simulink model "simulare"  (R2025b)
settings: Solver=VariableStepAuto  StartTime=0.0  StopTime=5  MaxStep=0.01  RelTol=1e-3
libraries: simulink x9
settings Model: Creator=alexolaru131  LastModifiedBy=alexolaru131

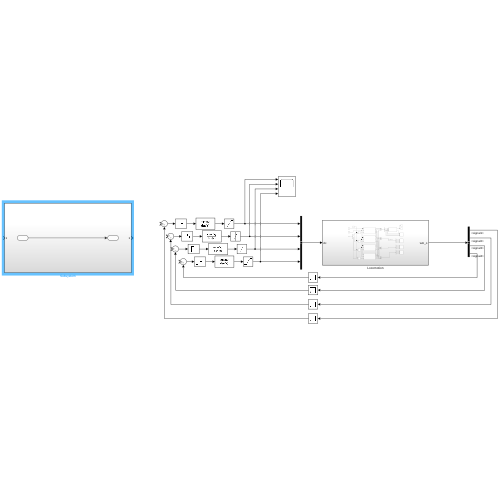
[thumbnail: Simulink's stored preview of the top-level diagram]
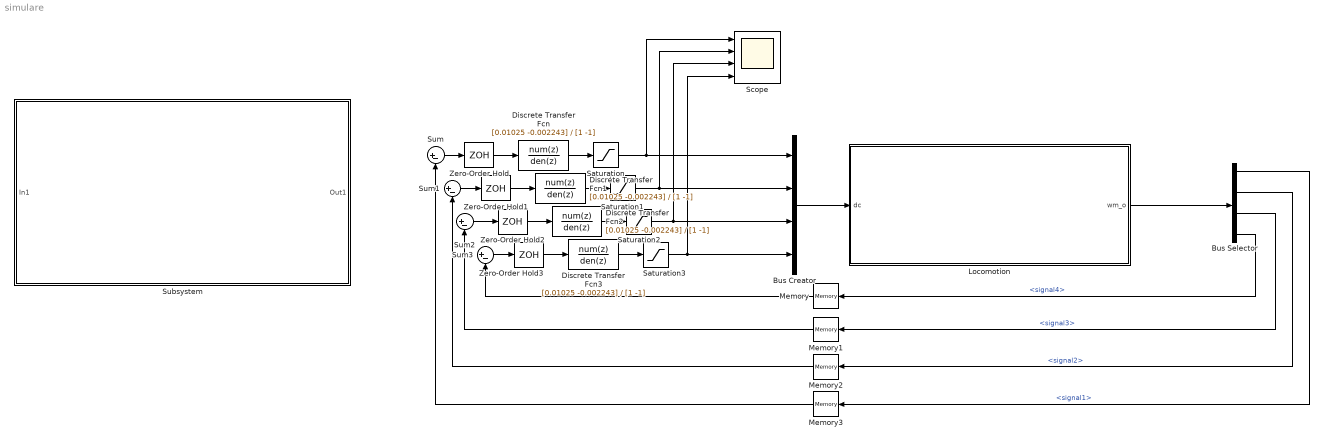
== system simulare ==
  Bus Creator : BusCreator  Inputs=4
  Bus Selector : BusSelector  OutputSignals=signal1,signal2,signal3,signal4
  Discrete Transfer Fcn{,1..3} (4 alike) : DiscreteTransferFcn  Numerator=[0.01025 -0.002243]  Denominator=[1 -1]
  Locomotion : Subsystem
  Memory{,1..3} (4 alike) : Memory
  Saturation{,1..3} (4 alike) : Saturate  UpperLimit=1  LowerLimit=0
  Scope : Scope  NumInputPorts=4
      settings: ActiveDisplayYMinimum=-1  ActiveDisplayYMaximum=1  DataLoggingVariableName=ScopeData4
  Subsystem : Subsystem
  Sum{,1..3} (4 alike) : Sum  Inputs=|+-
  Zero-Order Hold{,1..3} (4 alike) : ZeroOrderHold  SampleTime=0.1
  wires:
  Zero-Order Hold/1 -> Discrete Transfer Fcn/1
  Discrete Transfer Fcn/1 -> Saturation/1
  Sum/1 -> Zero-Order Hold/1
  Locomotion/1(wm_o) -> Bus Selector/1
  Bus Selector/1 -> Memory3/1  "<signal1>"
  Saturation/1 -> Scope/1, Bus Creator/1
  Saturation1/1 -> Bus Creator/2, Scope/2
  Discrete Transfer Fcn1/1 -> Saturation1/1
  Sum1/1 -> Zero-Order Hold1/1
  Zero-Order Hold1/1 -> Discrete Transfer Fcn1/1
  Bus Selector/2 -> Memory2/1  "<signal2>"
  Discrete Transfer Fcn2/1 -> Saturation2/1
  Zero-Order Hold2/1 -> Discrete Transfer Fcn2/1
  Saturation2/1 -> Bus Creator/3, Scope/3
  Sum2/1 -> Zero-Order Hold2/1
  Bus Selector/3 -> Memory1/1  "<signal3>"
  Discrete Transfer Fcn3/1 -> Saturation3/1
  Zero-Order Hold3/1 -> Discrete Transfer Fcn3/1
  Sum3/1 -> Zero-Order Hold3/1
  Saturation3/1 -> Bus Creator/4, Scope/4
  Bus Selector/4 -> Memory/1  "<signal4>"
  Memory/1 -> Sum3/2
  Memory1/1 -> Sum2/2
  Memory2/1 -> Sum1/2
  Memory3/1 -> Sum/2
  Bus Creator/1 -> Locomotion/1(dc)

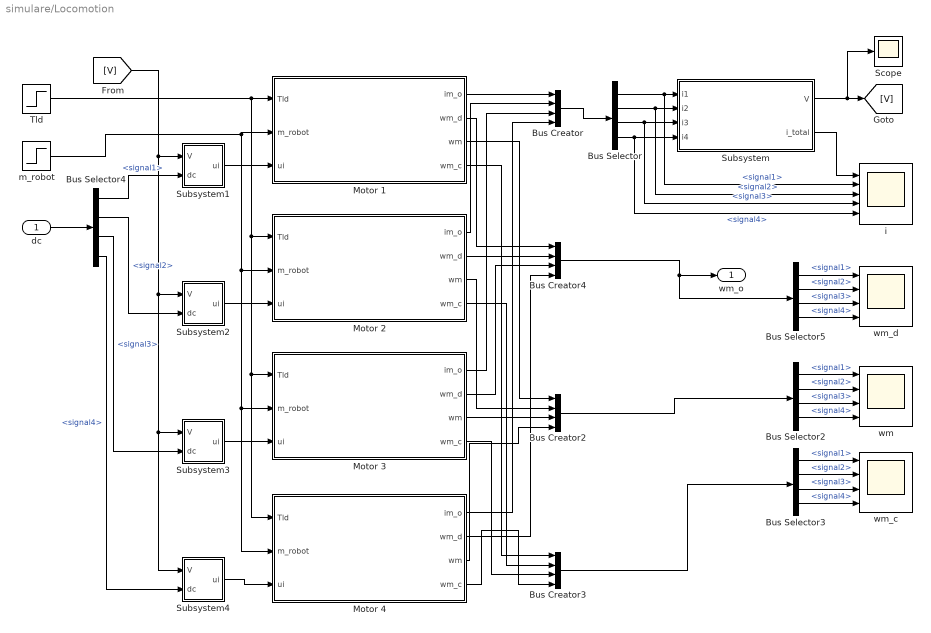
== system simulare/Locomotion ==
  dc : Inport
  Bus Creator{,2..4} (4 alike) : BusCreator  Inputs=4
  Bus Selector{,2..5} (5 alike) : BusSelector  OutputSignals=signal1,signal2,signal3,signal4
  Motor 1 : Subsystem
  Motor 2 : Subsystem
  Motor 3 : Subsystem
  Motor 4 : Subsystem
  Scope : Scope
      settings: ActiveDisplayYMinimum=-1  ActiveDisplayYMaximum=1
  Subsystem : Subsystem
  Subsystem1 : Subsystem
  Subsystem2 : Subsystem
  Subsystem3 : Subsystem
  Subsystem4 : Subsystem
  Tld : Step  Time=0  After=0.5  SampleTime=0
  i : Scope  NumInputPorts=5
      settings: ActiveDisplayYMinimum=-0.41798303299260658  ActiveDisplayYMaximum=3.1723127947753986
  m_robot : Step  Time=0  After=2000  SampleTime=0
  wm : Scope  NumInputPorts=4
      settings: ActiveDisplayYMinimum=-2.7499999999999996  ActiveDisplayYMaximum=24.75
  wm_c : Scope  NumInputPorts=4
      settings: ActiveDisplayYMinimum=-3.6972275501307741  ActiveDisplayYMaximum=33.275047951176973  DataLoggingVariableName=ScopeData3
  wm_d : Scope  NumInputPorts=4
      settings: ActiveDisplayYMinimum=-3.9543093339999862  ActiveDisplayYMaximum=35.588776352959464  DataLoggingVariableName=ScopeData2
  wm_o : Outport
  wires:
  Subsystem2/1(ui) -> Motor 2/3(ui)
  Subsystem1/1(ui) -> Motor 1/3(ui)
  Subsystem/2(i_total) -> i/1
  m_robot/1 -> Motor 1/2(m_robot), Motor 2/2(m_robot), Motor 3/2(m_robot), Motor 4/2(m_robot)
  Subsystem4/1(ui) -> Motor 4/3(ui)
  Tld/1 -> Motor 1/1(Tld), Motor 2/1(Tld), Motor 3/1(Tld), Motor 4/1(Tld)
  Subsystem3/1(ui) -> Motor 3/3(ui)
  Bus Creator/1 -> Bus Selector/1
  Bus Selector/1 -> i/2, Subsystem/1(i1)  "<signal1>"
  Bus Selector/2 -> Subsystem/2(i2), i/3  "<signal2>"
  Bus Selector/3 -> Subsystem/3(i3), i/4  "<signal3>"
  Bus Selector/4 -> Subsystem/4(i4), i/5  "<signal4>"
  Subsystem/1(V) -> Scope/1, [V]
  [V] -> Subsystem1/1(V), Subsystem2/1(V), Subsystem3/1(V), Subsystem4/1(V)
  Bus Selector2/2 -> wm/2  "<signal2>"
  Bus Selector2/1 -> wm/1  "<signal1>"
  Bus Selector2/3 -> wm/3  "<signal3>"
  Bus Selector2/4 -> wm/4  "<signal4>"
  Bus Creator2/1 -> Bus Selector2/1
  Bus Selector3/1 -> wm_c/1  "<signal1>"
  Bus Selector3/2 -> wm_c/2  "<signal2>"
  Bus Selector3/3 -> wm_c/3  "<signal3>"
  Bus Selector3/4 -> wm_c/4  "<signal4>"
  Bus Creator3/1 -> Bus Selector3/1
  Bus Selector5/4 -> wm_d/4  "<signal4>"
  Bus Creator4/1 -> Bus Selector5/1, wm_o/1
  Bus Selector5/2 -> wm_d/2  "<signal2>"
  Bus Selector5/3 -> wm_d/3  "<signal3>"
  Bus Selector5/1 -> wm_d/1  "<signal1>"
  Bus Selector4/1 -> Subsystem1/2(dc)  "<signal1>"
  Bus Selector4/2 -> Subsystem2/2(dc)  "<signal2>"
  Bus Selector4/3 -> Subsystem3/2(dc)  "<signal3>"
  Bus Selector4/4 -> Subsystem4/2(dc)  "<signal4>"
  dc/1 -> Bus Selector4/1
  Motor 1/1(im_o) -> Bus Creator/1
  Motor 2/1(im_o) -> Bus Creator/2
  Motor 3/1(im_o) -> Bus Creator/3
  Motor 4/1(im_o) -> Bus Creator/4
  Motor 1/2(wm_d) -> Bus Creator4/1
  Motor 2/2(wm_d) -> Bus Creator4/2
  Motor 3/2(wm_d) -> Bus Creator4/3
  Motor 4/2(wm_d) -> Bus Creator4/4
  Motor 1/3(wm) -> Bus Creator2/1
  Motor 2/3(wm) -> Bus Creator2/2
  Motor 3/3(wm) -> Bus Creator2/3
  Motor 4/3(wm) -> Bus Creator2/4
  Motor 1/4(wm_c) -> Bus Creator3/1
  Motor 2/4(wm_c) -> Bus Creator3/2
  Motor 3/4(wm_c) -> Bus Creator3/3
  Motor 4/4(wm_c) -> Bus Creator3/4

== system simulare/Subsystem ==
  In1 : Inport
  Out1 : Outport
  wires:
  In1/1 -> Out1/1

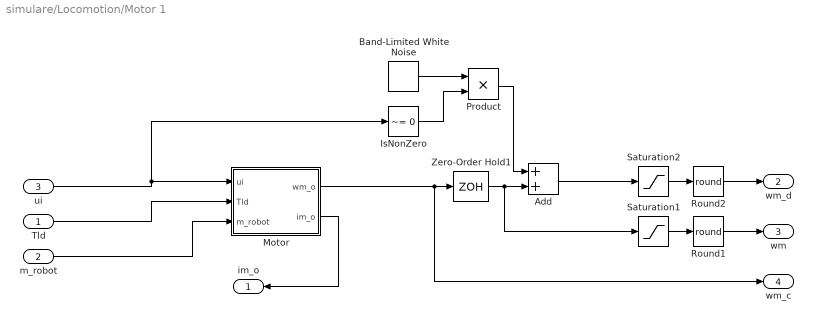
== system simulare/Locomotion/Motor 1 ==
  Tld : Inport
  m_robot : Inport  Port=2
  ui : Inport  Port=3
  Add : Sum
  Band-Limited White Noise : simulink/Sources/Band-Limited White Noise  Cov=[0.2]  Ts=0.1  seed=[1]
  IsNonZero : simulink/Logic and Bit Operations/Compare To Zero  relop=~=  OutDataTypeStr=boolean
      settings: LibrarySourceBlock=|
      | simulink/Quick Insert/Logic and Bit
      | Operations/IsNonZero
  Motor : Subsystem
  Product : Product
  Round1 : Rounding  Operator=round
  Round2 : Rounding  Operator=round
  Saturation1 : Saturate  UpperLimit=inf  LowerLimit=0
  Saturation2 : Saturate  UpperLimit=inf  LowerLimit=0
  Zero-Order Hold1 : ZeroOrderHold  SampleTime=0.1
  im_o : Outport
  wm_d : Outport  Port=2
  wm : Outport  Port=3
  wm_c : Outport  Port=4
  wires:
  Motor/2(im_o) -> im_o/1
  Tld/1 -> Motor/2(Tld)
  m_robot/1 -> Motor/3(m_robot)
  ui/1 -> IsNonZero/1, Motor/1(ui)
  Motor/1(wm_o) -> wm_c/1, Zero-Order Hold1/1
  IsNonZero/1 -> Product/2
  Product/1 -> Add/1
  Add/1 -> Saturation2/1
  Zero-Order Hold1/1 -> Saturation1/1, Add/2
  Saturation1/1 -> Round1/1
  Round1/1 -> wm/1
  Band-Limited White Noise/1 -> Product/1
  Round2/1 -> wm_d/1
  Saturation2/1 -> Round2/1

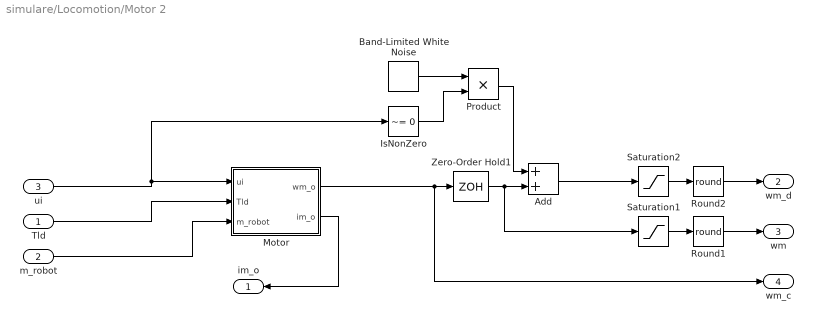
== system simulare/Locomotion/Motor 2 ==
  Tld : Inport
  m_robot : Inport  Port=2
  ui : Inport  Port=3
  Add : Sum
  Band-Limited White Noise : simulink/Sources/Band-Limited White Noise  Cov=[0.2]  Ts=0.1  seed=[2]
  IsNonZero : simulink/Logic and Bit Operations/Compare To Zero  relop=~=  OutDataTypeStr=boolean
      settings: LibrarySourceBlock=|
      | simulink/Quick Insert/Logic and Bit
      | Operations/IsNonZero
  Motor : Subsystem
  Product : Product
  Round1 : Rounding  Operator=round
  Round2 : Rounding  Operator=round
  Saturation1 : Saturate  UpperLimit=inf  LowerLimit=0
  Saturation2 : Saturate  UpperLimit=inf  LowerLimit=0
  Zero-Order Hold1 : ZeroOrderHold  SampleTime=0.1
  im_o : Outport
  wm_d : Outport  Port=2
  wm : Outport  Port=3
  wm_c : Outport  Port=4
  wires:
  Motor/2(im_o) -> im_o/1
  Tld/1 -> Motor/2(Tld)
  m_robot/1 -> Motor/3(m_robot)
  ui/1 -> IsNonZero/1, Motor/1(ui)
  Motor/1(wm_o) -> wm_c/1, Zero-Order Hold1/1
  IsNonZero/1 -> Product/2
  Product/1 -> Add/1
  Add/1 -> Saturation2/1
  Zero-Order Hold1/1 -> Saturation1/1, Add/2
  Saturation1/1 -> Round1/1
  Round1/1 -> wm/1
  Band-Limited White Noise/1 -> Product/1
  Round2/1 -> wm_d/1
  Saturation2/1 -> Round2/1

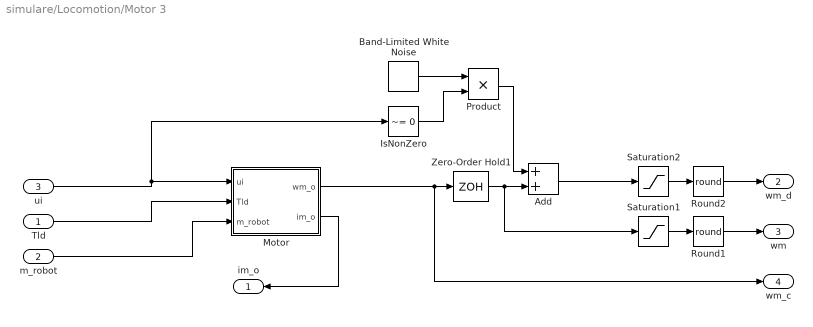
== system simulare/Locomotion/Motor 3 ==
  Tld : Inport
  m_robot : Inport  Port=2
  ui : Inport  Port=3
  Add : Sum
  Band-Limited White Noise : simulink/Sources/Band-Limited White Noise  Cov=[0.2]  Ts=0.1  seed=[3]
  IsNonZero : simulink/Logic and Bit Operations/Compare To Zero  relop=~=  OutDataTypeStr=boolean
      settings: LibrarySourceBlock=|
      | simulink/Quick Insert/Logic and Bit
      | Operations/IsNonZero
  Motor : Subsystem
  Product : Product
  Round1 : Rounding  Operator=round
  Round2 : Rounding  Operator=round
  Saturation1 : Saturate  UpperLimit=inf  LowerLimit=0
  Saturation2 : Saturate  UpperLimit=inf  LowerLimit=0
  Zero-Order Hold1 : ZeroOrderHold  SampleTime=0.1
  im_o : Outport
  wm_d : Outport  Port=2
  wm : Outport  Port=3
  wm_c : Outport  Port=4
  wires:
  Motor/2(im_o) -> im_o/1
  Tld/1 -> Motor/2(Tld)
  m_robot/1 -> Motor/3(m_robot)
  ui/1 -> IsNonZero/1, Motor/1(ui)
  Motor/1(wm_o) -> wm_c/1, Zero-Order Hold1/1
  IsNonZero/1 -> Product/2
  Product/1 -> Add/1
  Add/1 -> Saturation2/1
  Zero-Order Hold1/1 -> Saturation1/1, Add/2
  Saturation1/1 -> Round1/1
  Round1/1 -> wm/1
  Band-Limited White Noise/1 -> Product/1
  Round2/1 -> wm_d/1
  Saturation2/1 -> Round2/1

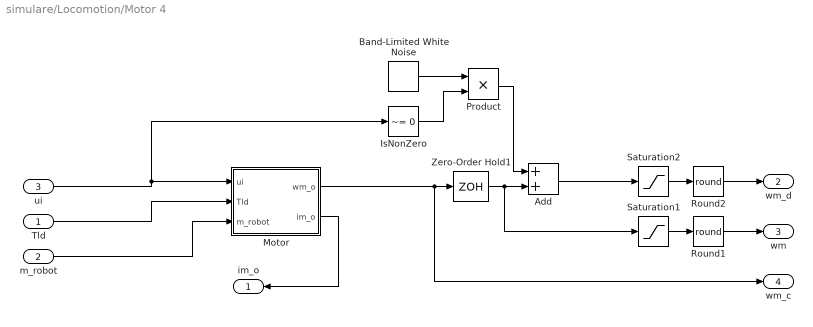
== system simulare/Locomotion/Motor 4 ==
  Tld : Inport
  m_robot : Inport  Port=2
  ui : Inport  Port=3
  Add : Sum
  Band-Limited White Noise : simulink/Sources/Band-Limited White Noise  Cov=[0.2]  Ts=0.1  seed=[4]
  IsNonZero : simulink/Logic and Bit Operations/Compare To Zero  relop=~=  OutDataTypeStr=boolean
      settings: LibrarySourceBlock=|
      | simulink/Quick Insert/Logic and Bit
      | Operations/IsNonZero
  Motor : Subsystem
  Product : Product
  Round1 : Rounding  Operator=round
  Round2 : Rounding  Operator=round
  Saturation1 : Saturate  UpperLimit=inf  LowerLimit=0
  Saturation2 : Saturate  UpperLimit=inf  LowerLimit=0
  Zero-Order Hold1 : ZeroOrderHold  SampleTime=0.1
  im_o : Outport
  wm_d : Outport  Port=2
  wm : Outport  Port=3
  wm_c : Outport  Port=4
  wires:
  Motor/2(im_o) -> im_o/1
  Tld/1 -> Motor/2(Tld)
  m_robot/1 -> Motor/3(m_robot)
  ui/1 -> IsNonZero/1, Motor/1(ui)
  Motor/1(wm_o) -> wm_c/1, Zero-Order Hold1/1
  IsNonZero/1 -> Product/2
  Product/1 -> Add/1
  Add/1 -> Saturation2/1
  Zero-Order Hold1/1 -> Saturation1/1, Add/2
  Saturation1/1 -> Round1/1
  Round1/1 -> wm/1
  Band-Limited White Noise/1 -> Product/1
  Round2/1 -> wm_d/1
  Saturation2/1 -> Round2/1

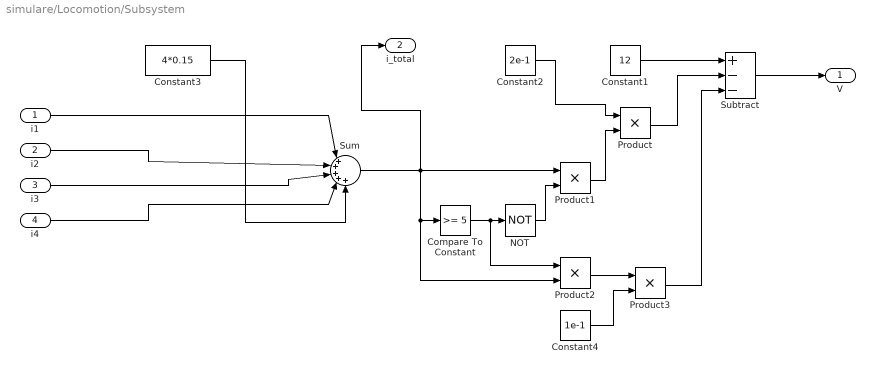
== system simulare/Locomotion/Subsystem ==
  i1 : Inport
  i2 : Inport  Port=2
  i3 : Inport  Port=3
  i4 : Inport  Port=4
  Compare To Constant : simulink/Logic and Bit Operations/Compare To Constant  relop=>=  const=5  OutDataTypeStr=boolean  ZeroCross=off
  Constant1 : Constant  Value=12
  Constant2 : Constant  Value=2e-1
  Constant3 : Constant  Value=4*0.15
  Constant4 : Constant  Value=1e-1
  NOT : Logic  Operator=NOT  IconShape=distinctive  AllPortsSameDT=off  OutDataTypeStr=boolean
  Product{,1..3} (4 alike) : Product
  Subtract : Sum  Inputs=+--
  Sum : Sum  Inputs=|+++++
  V : Outport
  i_total : Outport  Port=2
  wires:
  Constant2/1 -> Product/1
  Product/1 -> Subtract/2
  Sum/1 -> Product2/2, Compare To Constant/1, Product1/1, i_total/1
  Constant3/1 -> Sum/5
  Constant1/1 -> Subtract/1
  i1/1 -> Sum/1
  i2/1 -> Sum/2
  i3/1 -> Sum/3
  i4/1 -> Sum/4
  Subtract/1 -> V/1
  Compare To Constant/1 -> Product2/1, NOT/1
  NOT/1 -> Product1/2
  Product1/1 -> Product/2
  Product2/1 -> Product3/1
  Product3/1 -> Subtract/3
  Constant4/1 -> Product3/2

== system simulare/Locomotion/Subsystem1 ==
  V : Inport
  dc : Inport  Port=2
  Add : Sum  Inputs=+-
  Constant : Constant  Value=1.2782
  Product : Product
  ui : Outport
  wires:
  Add/1 -> Product/1
  V/1 -> Add/1
  dc/1 -> Product/2
  Constant/1 -> Add/2
  Product/1 -> ui/1

== system simulare/Locomotion/Subsystem2 ==
  V : Inport
  dc : Inport  Port=2
  Add : Sum  Inputs=+-
  Constant : Constant  Value=1.2782
  Product : Product
  ui : Outport
  wires:
  Add/1 -> Product/1
  V/1 -> Add/1
  dc/1 -> Product/2
  Constant/1 -> Add/2
  Product/1 -> ui/1

== system simulare/Locomotion/Subsystem3 ==
  V : Inport
  dc : Inport  Port=2
  Add : Sum  Inputs=+-
  Constant : Constant  Value=1.2782
  Product : Product
  ui : Outport
  wires:
  Add/1 -> Product/1
  V/1 -> Add/1
  dc/1 -> Product/2
  Constant/1 -> Add/2
  Product/1 -> ui/1

== system simulare/Locomotion/Subsystem4 ==
  V : Inport
  dc : Inport  Port=2
  Add : Sum  Inputs=+-
  Constant : Constant  Value=1.2782
  Product : Product
  ui : Outport
  wires:
  Add/1 -> Product/1
  V/1 -> Add/1
  dc/1 -> Product/2
  Constant/1 -> Add/2
  Product/1 -> ui/1

== system simulare/Locomotion/Motor 1/Motor ==
  ui : Inport
  Tld : Inport  Port=2
  m_robot : Inport  Port=3
  Electric : Subsystem
  Mecanic : Subsystem
  wm_o : Outport
  im_o : Outport  Port=2
  wires:
  Tld/1 -> Mecanic/2(Tld)
  Mecanic/1(wm_o) -> wm_o/1, Electric/3(wm), Mecanic/3(wm_i)
  Electric/1(im_o) -> im_o/1, Mecanic/1(im_i), Electric/2(im_i)
  m_robot/1 -> Mecanic/4(m_robot)
  ui/1 -> Electric/1(ui)

== system simulare/Locomotion/Motor 2/Motor ==
  ui : Inport
  Tld : Inport  Port=2
  m_robot : Inport  Port=3
  Electric : Subsystem
  Mecanic : Subsystem
  wm_o : Outport
  im_o : Outport  Port=2
  wires:
  Tld/1 -> Mecanic/2(Tld)
  Mecanic/1(wm_o) -> wm_o/1, Electric/3(wm), Mecanic/3(wm_i)
  Electric/1(im_o) -> im_o/1, Mecanic/1(im_i), Electric/2(im_i)
  m_robot/1 -> Mecanic/4(m_robot)
  ui/1 -> Electric/1(ui)

== system simulare/Locomotion/Motor 3/Motor ==
  ui : Inport
  Tld : Inport  Port=2
  m_robot : Inport  Port=3
  Electric : Subsystem
  Mecanic : Subsystem
  wm_o : Outport
  im_o : Outport  Port=2
  wires:
  Tld/1 -> Mecanic/2(Tld)
  Mecanic/1(wm_o) -> wm_o/1, Electric/3(wm), Mecanic/3(wm_i)
  Electric/1(im_o) -> im_o/1, Mecanic/1(im_i), Electric/2(im_i)
  m_robot/1 -> Mecanic/4(m_robot)
  ui/1 -> Electric/1(ui)

== system simulare/Locomotion/Motor 4/Motor ==
  ui : Inport
  Tld : Inport  Port=2
  m_robot : Inport  Port=3
  Electric : Subsystem
  Mecanic : Subsystem
  wm_o : Outport
  im_o : Outport  Port=2
  wires:
  Tld/1 -> Mecanic/2(Tld)
  Mecanic/1(wm_o) -> wm_o/1, Electric/3(wm), Mecanic/3(wm_i)
  Electric/1(im_o) -> im_o/1, Mecanic/1(im_i), Electric/2(im_i)
  m_robot/1 -> Mecanic/4(m_robot)
  ui/1 -> Electric/1(ui)

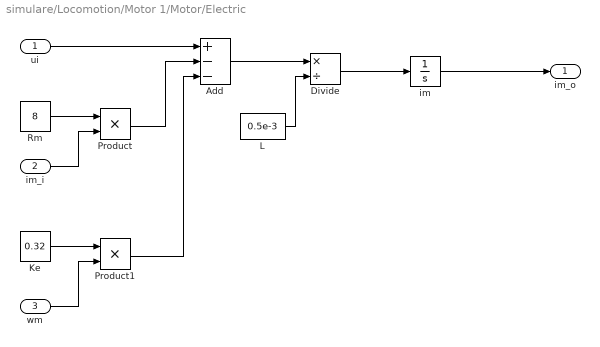
== system simulare/Locomotion/Motor 1/Motor/Electric ==
  ui : Inport
  im_i : Inport  Port=2
  wm : Inport  Port=3
  Add : Sum  Inputs=+--
  Divide : Product  Inputs=*/
  Ke : Constant  Value=0.32
  L : Constant  Value=0.5e-3
  Product : Product
  Product1 : Product
  Rm : Constant  Value=8
  im : Integrator  LimitOutput=on  UpperSaturationLimit=5  LowerSaturationLimit=0
  im_o : Outport
  wires:
  im_i/1 -> Product/2
  Rm/1 -> Product/1
  ui/1 -> Add/1
  Divide/1 -> im/1
  wm/1 -> Product1/2
  Ke/1 -> Product1/1
  Product1/1 -> Add/3
  L/1 -> Divide/2
  Add/1 -> Divide/1
  Product/1 -> Add/2
  im/1 -> im_o/1

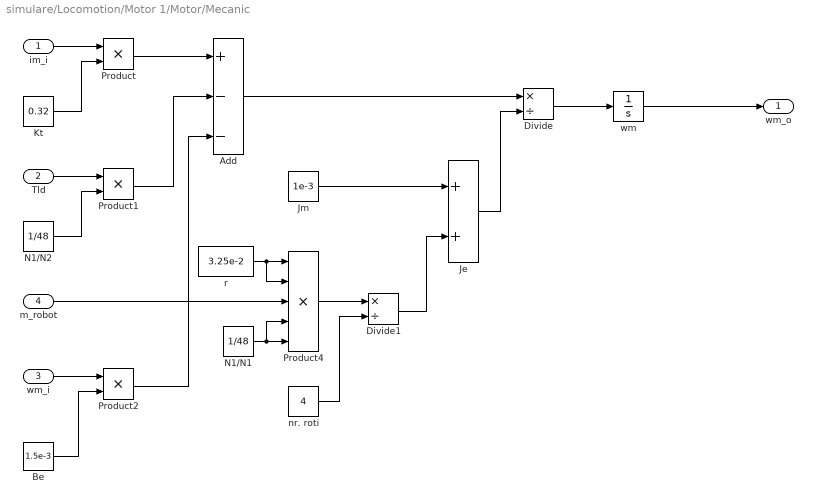
== system simulare/Locomotion/Motor 1/Motor/Mecanic ==
  im_i : Inport
  Tld : Inport  Port=2
  wm_i : Inport  Port=3
  m_robot : Inport  Port=4
  Add : Sum  Inputs=+--
  Be : Constant  Value=1.5e-3
  Divide : Product  Inputs=*/
  Divide1 : Product  Inputs=*/
  Je : Sum
  Jm : Constant  Value=1e-3
  Kt : Constant  Value=0.32
  N1/N1 : Constant  Value=1/48
  N1/N2 : Constant  Value=1/48
  Product : Product
  Product1 : Product
  Product2 : Product
  Product4 : Product  Inputs=5
  nr. roti : Constant  Value=4
  r : Constant  Value=3.25e-2
  wm : Integrator  UpperSaturationLimit=24  LowerSaturationLimit=0
  wm_o : Outport
  wires:
  Add/1 -> Divide/1
  Tld/1 -> Product1/1
  Product2/1 -> Add/3
  im_i/1 -> Product/1
  Product/1 -> Add/1
  m_robot/1 -> Product4/3
  N1/N2/1 -> Product1/2
  Kt/1 -> Product/2
  wm_i/1 -> Product2/1
  Jm/1 -> Je/1
  r/1 -> Product4/2, Product4/1
  Je/1 -> Divide/2
  Be/1 -> Product2/2
  Divide/1 -> wm/1
  Product1/1 -> Add/2
  N1/N1/1 -> Product4/5, Product4/4
  Product4/1 -> Divide1/1
  nr. roti/1 -> Divide1/2
  Divide1/1 -> Je/2
  wm/1 -> wm_o/1

== system simulare/Locomotion/Motor 2/Motor/Electric ==
  ui : Inport
  im_i : Inport  Port=2
  wm : Inport  Port=3
  Add : Sum  Inputs=+--
  Divide : Product  Inputs=*/
  Ke : Constant  Value=0.32
  L : Constant  Value=0.5e-3
  Product : Product
  Product1 : Product
  Rm : Constant  Value=8
  im : Integrator  LimitOutput=on  UpperSaturationLimit=5  LowerSaturationLimit=0
  im_o : Outport
  wires:
  im_i/1 -> Product/2
  Rm/1 -> Product/1
  ui/1 -> Add/1
  Divide/1 -> im/1
  wm/1 -> Product1/2
  Ke/1 -> Product1/1
  Product1/1 -> Add/3
  L/1 -> Divide/2
  Add/1 -> Divide/1
  Product/1 -> Add/2
  im/1 -> im_o/1

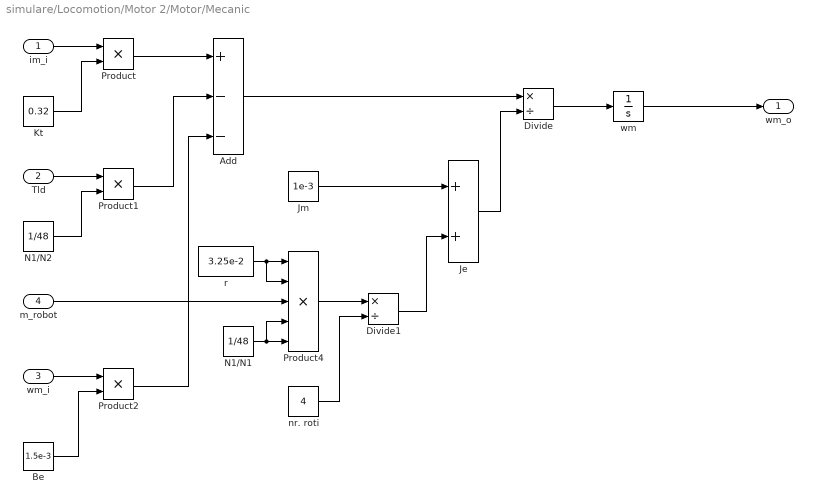
== system simulare/Locomotion/Motor 2/Motor/Mecanic ==
  im_i : Inport
  Tld : Inport  Port=2
  wm_i : Inport  Port=3
  m_robot : Inport  Port=4
  Add : Sum  Inputs=+--
  Be : Constant  Value=1.5e-3
  Divide : Product  Inputs=*/
  Divide1 : Product  Inputs=*/
  Je : Sum
  Jm : Constant  Value=1e-3
  Kt : Constant  Value=0.32
  N1/N1 : Constant  Value=1/48
  N1/N2 : Constant  Value=1/48
  Product : Product
  Product1 : Product
  Product2 : Product
  Product4 : Product  Inputs=5
  nr. roti : Constant  Value=4
  r : Constant  Value=3.25e-2
  wm : Integrator  UpperSaturationLimit=24  LowerSaturationLimit=0
  wm_o : Outport
  wires:
  Add/1 -> Divide/1
  Tld/1 -> Product1/1
  Product2/1 -> Add/3
  im_i/1 -> Product/1
  Product/1 -> Add/1
  m_robot/1 -> Product4/3
  N1/N2/1 -> Product1/2
  Kt/1 -> Product/2
  wm_i/1 -> Product2/1
  Jm/1 -> Je/1
  r/1 -> Product4/2, Product4/1
  Je/1 -> Divide/2
  Be/1 -> Product2/2
  Divide/1 -> wm/1
  Product1/1 -> Add/2
  N1/N1/1 -> Product4/5, Product4/4
  Product4/1 -> Divide1/1
  nr. roti/1 -> Divide1/2
  Divide1/1 -> Je/2
  wm/1 -> wm_o/1

== system simulare/Locomotion/Motor 3/Motor/Electric ==
  ui : Inport
  im_i : Inport  Port=2
  wm : Inport  Port=3
  Add : Sum  Inputs=+--
  Divide : Product  Inputs=*/
  Ke : Constant  Value=0.32
  L : Constant  Value=0.5e-3
  Product : Product
  Product1 : Product
  Rm : Constant  Value=8
  im : Integrator  LimitOutput=on  UpperSaturationLimit=5  LowerSaturationLimit=0
  im_o : Outport
  wires:
  im_i/1 -> Product/2
  Rm/1 -> Product/1
  ui/1 -> Add/1
  Divide/1 -> im/1
  wm/1 -> Product1/2
  Ke/1 -> Product1/1
  Product1/1 -> Add/3
  L/1 -> Divide/2
  Add/1 -> Divide/1
  Product/1 -> Add/2
  im/1 -> im_o/1

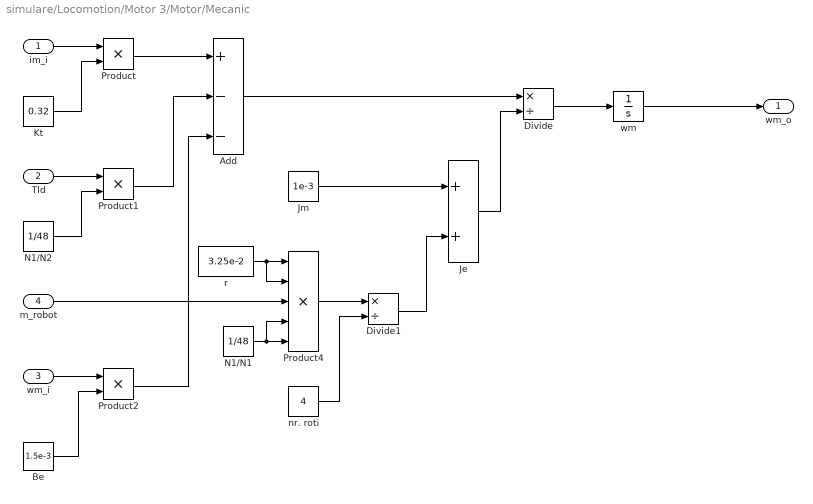
== system simulare/Locomotion/Motor 3/Motor/Mecanic ==
  im_i : Inport
  Tld : Inport  Port=2
  wm_i : Inport  Port=3
  m_robot : Inport  Port=4
  Add : Sum  Inputs=+--
  Be : Constant  Value=1.5e-3
  Divide : Product  Inputs=*/
  Divide1 : Product  Inputs=*/
  Je : Sum
  Jm : Constant  Value=1e-3
  Kt : Constant  Value=0.32
  N1/N1 : Constant  Value=1/48
  N1/N2 : Constant  Value=1/48
  Product : Product
  Product1 : Product
  Product2 : Product
  Product4 : Product  Inputs=5
  nr. roti : Constant  Value=4
  r : Constant  Value=3.25e-2
  wm : Integrator  UpperSaturationLimit=24  LowerSaturationLimit=0
  wm_o : Outport
  wires:
  Add/1 -> Divide/1
  Tld/1 -> Product1/1
  Product2/1 -> Add/3
  im_i/1 -> Product/1
  Product/1 -> Add/1
  m_robot/1 -> Product4/3
  N1/N2/1 -> Product1/2
  Kt/1 -> Product/2
  wm_i/1 -> Product2/1
  Jm/1 -> Je/1
  r/1 -> Product4/2, Product4/1
  Je/1 -> Divide/2
  Be/1 -> Product2/2
  Divide/1 -> wm/1
  Product1/1 -> Add/2
  N1/N1/1 -> Product4/5, Product4/4
  Product4/1 -> Divide1/1
  nr. roti/1 -> Divide1/2
  Divide1/1 -> Je/2
  wm/1 -> wm_o/1

== system simulare/Locomotion/Motor 4/Motor/Electric ==
  ui : Inport
  im_i : Inport  Port=2
  wm : Inport  Port=3
  Add : Sum  Inputs=+--
  Divide : Product  Inputs=*/
  Ke : Constant  Value=0.32
  L : Constant  Value=0.5e-3
  Product : Product
  Product1 : Product
  Rm : Constant  Value=8
  im : Integrator  LimitOutput=on  UpperSaturationLimit=5  LowerSaturationLimit=0
  im_o : Outport
  wires:
  im_i/1 -> Product/2
  Rm/1 -> Product/1
  ui/1 -> Add/1
  Divide/1 -> im/1
  wm/1 -> Product1/2
  Ke/1 -> Product1/1
  Product1/1 -> Add/3
  L/1 -> Divide/2
  Add/1 -> Divide/1
  Product/1 -> Add/2
  im/1 -> im_o/1

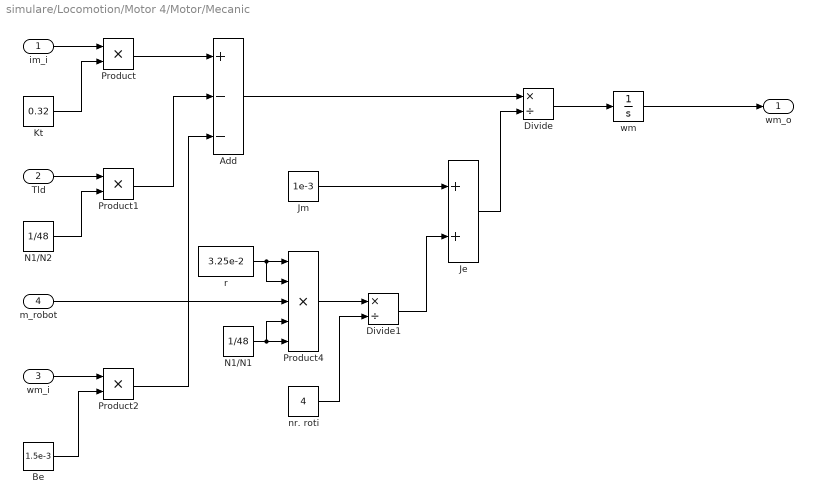
== system simulare/Locomotion/Motor 4/Motor/Mecanic ==
  im_i : Inport
  Tld : Inport  Port=2
  wm_i : Inport  Port=3
  m_robot : Inport  Port=4
  Add : Sum  Inputs=+--
  Be : Constant  Value=1.5e-3
  Divide : Product  Inputs=*/
  Divide1 : Product  Inputs=*/
  Je : Sum
  Jm : Constant  Value=1e-3
  Kt : Constant  Value=0.32
  N1/N1 : Constant  Value=1/48
  N1/N2 : Constant  Value=1/48
  Product : Product
  Product1 : Product
  Product2 : Product
  Product4 : Product  Inputs=5
  nr. roti : Constant  Value=4
  r : Constant  Value=3.25e-2
  wm : Integrator  UpperSaturationLimit=24  LowerSaturationLimit=0
  wm_o : Outport
  wires:
  Add/1 -> Divide/1
  Tld/1 -> Product1/1
  Product2/1 -> Add/3
  im_i/1 -> Product/1
  Product/1 -> Add/1
  m_robot/1 -> Product4/3
  N1/N2/1 -> Product1/2
  Kt/1 -> Product/2
  wm_i/1 -> Product2/1
  Jm/1 -> Je/1
  r/1 -> Product4/2, Product4/1
  Je/1 -> Divide/2
  Be/1 -> Product2/2
  Divide/1 -> wm/1
  Product1/1 -> Add/2
  N1/N1/1 -> Product4/5, Product4/4
  Product4/1 -> Divide1/1
  nr. roti/1 -> Divide1/2
  Divide1/1 -> Je/2
  wm/1 -> wm_o/1
